simulink model "Xcvr_SSB_AM_2p5"  (Simulink 7.4)
settings: Solver=VariableStepDiscrete  SolverMode=SingleTasking  StartTime=0.0  StopTime=10  RelTol=1e-3
PreLoadFcn:
  | Fs=80e6;
  | 
  | phee=da_rom();
  | [phee_1,phee_2]=da_i2_rom();
  | 
  | Dcic=64;       % CIC decimation
  | Dfac=128;    % following DA filter decimation
  | N = 6;           %       (2^(N+1))=Dfac
  | Daudio=Dcic*Dfac;
  | Faudio=Fs/Daudio;
  | 
  | load info_filt_ssb_4
  | load Serial_Intfc_Stream_5
  | 
  | % AGC related
  | x=0.5:1/256:(1-1/256);
  | addr=(x-0.5)*256;
  | y=1./x;
undefined symbols (not defined in the file): Serial_Interface, ssb_coef, xlipgetpartsetting
libraries: xbsIndex_r4 x1305, dspsrcs4 x5, simulink x2, dspsigops x2, dspsnks4 x1
(part 7 of 11)

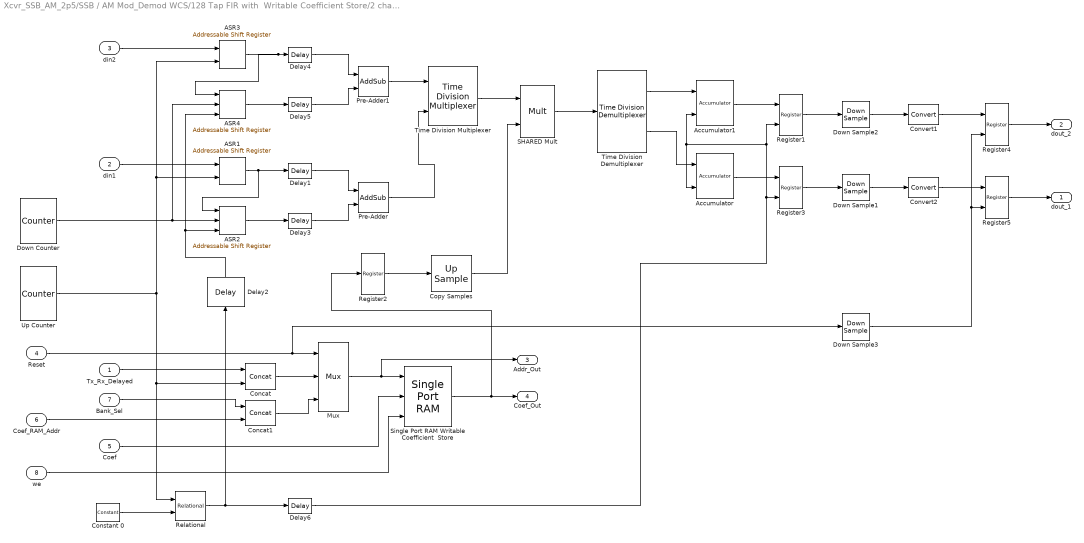
== system Xcvr_SSB_AM_2p5/SSB / AM Mod_Demod WCS/128 Tap FIR with  Writable Coefficient Store/2 channel (IQ)  SHARED MPY MAC with Writable Coefficient Store ==
  Tx_Rx_Delayed : Inport  OutDataType=sfix(16)  OutScaling=2^0
  din1 : Inport  Port=2  OutDataType=sfix(16)  OutScaling=2^0
  din2 : Inport  Port=3  OutDataType=sfix(16)  OutScaling=2^0
  Reset : Inport  Port=4  OutDataType=sfix(16)  OutScaling=2^0
  Coef : Inport  Port=5  OutDataType=sfix(16)  OutScaling=2^0
  Coef_RAM_Addr : Inport  Port=6  OutDataType=sfix(16)  OutScaling=2^0
  Bank_Sel : Inport  Port=7  OutDataType=sfix(16)  OutScaling=2^0
  we : Inport  Port=8  OutDataType=sfix(16)  OutScaling=2^0
  ASR1 : xbsIndex_r4/Addressable Shift Register  infer_latency=on  depth=2  initVector=0  en=off  dbl_ovrd=off  use_behavioral_HDL=off  use_rpm=off  block_type=addrsr
      settings: infoedit="Delay of configurable length.  Any element in the delay line can be addressed and driven onto the output port.<P><P>Hardware notes: Implemented using SRL16s.  If a Virtex-II device is used, multiple SRLC16s are cascaded together."  xl_area=[0, 0, 0, 0, 0, 0, 0]  block_version=VER_STRING_GOES_HERE
  ASR2 : xbsIndex_r4/Addressable Shift Register  infer_latency=on  depth=2  initVector=0  en=on  dbl_ovrd=off  use_behavioral_HDL=off  use_rpm=off  block_type=addrsr
      settings: infoedit="Delay of configurable length.  Any element in the delay line can be addressed and driven onto the output port.<P><P>Hardware notes: Implemented using SRL16s.  If a Virtex-II device is used, multiple SRLC16s are cascaded together."  xl_area=[0, 0, 0, 0, 0, 0, 0]  block_version=VER_STRING_GOES_HERE
  ASR3 : xbsIndex_r4/Addressable Shift Register  infer_latency=on  depth=2  initVector=0  en=off  dbl_ovrd=off  use_behavioral_HDL=off  use_rpm=off  block_type=addrsr
      settings: infoedit="Delay of configurable length.  Any element in the delay line can be addressed and driven onto the output port.<P><P>Hardware notes: Implemented using SRL16s.  If a Virtex-II device is used, multiple SRLC16s are cascaded together."  xl_area=[0, 0, 0, 0, 0, 0, 0]  block_version=VER_STRING_GOES_HERE
  ASR4 : xbsIndex_r4/Addressable Shift Register  infer_latency=on  depth=2  initVector=0  en=on  dbl_ovrd=off  use_behavioral_HDL=off  use_rpm=off  block_type=addrsr
      settings: infoedit="Delay of configurable length.  Any element in the delay line can be addressed and driven onto the output port.<P><P>Hardware notes: Implemented using SRL16s.  If a Virtex-II device is used, multiple SRLC16s are cascaded together."  xl_area=[0, 0, 0, 0, 0, 0, 0]  block_version=VER_STRING_GOES_HERE
  Accumulator : xbsIndex_r4/Accumulator  operation=Add  n_bits=ceil(log2(max(1,sum(abs(coef*2^coef_bin_pt)))))+smpl_n_bits + 1  overflow=Wrap  scale=1  rst=on  hasbypass=on  en=off  dbl_ovrd=off  use_behavioral_HDL=on  implementation=Fabric  block_type=accum
      settings: infoedit="Adder or subtractor-based accumulator.   Output type and binary point position match the input.<P><P>Hardware notes: When \"Reinitialize with Input 'b' on Reset\" is selected, the accumulator is forced to run at the system rate even if the input 'b' is running at a slower rate."  xl_area=[0, 0, 0, 0, 0, 0, 0]  block_version=VER_STRING_GOES_HERE
  Accumulator1 : xbsIndex_r4/Accumulator  operation=Add  n_bits=ceil(log2(max(1,sum(abs(coef*2^coef_bin_pt)))))+smpl_n_bits + 1  overflow=Wrap  scale=1  rst=on  hasbypass=on  en=off  dbl_ovrd=off  use_behavioral_HDL=on  implementation=Fabric  block_type=accum
      settings: infoedit="Adder or subtractor-based accumulator.   Output type and binary point position match the input.<P><P>Hardware notes: When \"Reinitialize with Input 'b' on Reset\" is selected, the accumulator is forced to run at the system rate even if the input 'b' is running at a slower rate."  xl_area=[0, 0, 0, 0, 0, 0, 0]  block_version=VER_STRING_GOES_HERE
  Concat : xbsIndex_r4/Concat  num_inputs=2  dbl_ovrd=off  block_type=concat
      settings: block_version=12.2
  Concat1 : xbsIndex_r4/Concat  num_inputs=2  dbl_ovrd=off  block_type=concat
      settings: block_version=12.2
  Constant 0 : xbsIndex_r4/Constant  arith_type=Unsigned  const=0  n_bits=1  bin_pt=0  explicit_period=off  period=1  equ=P=C  opselect=C  inp2=PCIN>>17  opr=+  inp1=P  carry=CIN  dbl_ovrd=off  block_type=constant
      settings: block_version=VER_STRING_GOES_HERE
  Convert1 : xbsIndex_r4/Convert  arith_type="Signed  (2's comp)"  n_bits=18  bin_pt=17  quantization="Round  (unbiased: +/- Inf)"  overflow=Wrap  en=off  latency=0  dbl_ovrd=off  pipeline=off  block_type=convert
      settings: block_version=9.2.00
  Convert2 : xbsIndex_r4/Convert  arith_type="Signed  (2's comp)"  n_bits=18  bin_pt=17  quantization="Round  (unbiased: +/- Inf)"  overflow=Wrap  en=off  latency=0  dbl_ovrd=off  pipeline=off  block_type=convert
      settings: block_version=9.2.00
  Copy Samples : xbsIndex_r4/Up Sample  sample_ratio=2  copy_samples=on  en=off  latency=0  dbl_ovrd=off  block_type=usamp
      settings: block_version=12.1
  Delay{1,3..5} (4 alike) : xbsIndex_r4/Delay  en=off  latency=1  dbl_ovrd=off  reg_retiming=off  block_type=delay
      settings: infoedit="Delay line having  configurable length.<P><P>Hardware notes: A delay line is a chain, each link of which is an SRL16 followed by a flip-flop. If register retiming is enabled, the delay line is a chain of flip-flops."  xl_area=[0, 0, 0, 0, 0, 0, 0]  block_version=VER_STRING_GOES_HERE
  Delay2 : xbsIndex_r4/Delay  en=off  latency=(length(coef)/2)-2  dbl_ovrd=off  reg_retiming=off  block_type=delay
      settings: infoedit="Delay line having  configurable length.<P><P>Hardware notes: A delay line is a chain, each link of which is an SRL16 followed by a flip-flop. If register retiming is enabled, the delay line is a chain of flip-flops."  xl_area=[0, 0, 0, 0, 0, 0, 0]  block_version=VER_STRING_GOES_HERE
  Delay6 : xbsIndex_r4/Delay  en=off  latency=3  dbl_ovrd=off  reg_retiming=off  block_type=delay
      settings: xl_area=[0, 0, 0, 0, 0, 0, 0]  block_version=VER_STRING_GOES_HERE
  Down Counter : xbsIndex_r4/Counter  cnt_type=Count Limited  cnt_to=0  operation=Down  start_count=(length(coef)/2)-1  cnt_by_val=1  arith_type=Unsigned  n_bits=ceil(log2(length(coef)/2))  bin_pt=0  load_pin=off  rst=off  en=off  explicit_period=on  period=smpl_period/(length(coef)/2)  dbl_ovrd=off  use_behavioral_HDL=off  implementation=Fabric  use_rpm=off  block_type=counter
      settings: xl_area=[0, 0, 0, 0, 0, 0, 0]  block_version=VER_STRING_GOES_HERE
  Down Sample1 : xbsIndex_r4/Down Sample  sample_ratio=length(coef)/2  sample_phase="Last Value of Frame  (most efficient)"  en=off  latency=1  dbl_ovrd=off  block_type=dsamp
      settings: xl_area=[0, 0, 0, 0, 0, 0, 0]  block_version=VER_STRING_GOES_HERE
  Down Sample2 : xbsIndex_r4/Down Sample  sample_ratio=length(coef)/2  sample_phase="Last Value of Frame  (most efficient)"  en=off  latency=1  dbl_ovrd=off  block_type=dsamp
      settings: xl_area=[0, 0, 0, 0, 0, 0, 0]  block_version=VER_STRING_GOES_HERE
  Down Sample3 : xbsIndex_r4/Down Sample  sample_ratio=4  sample_phase="Last Value of Frame  (most efficient)"  en=off  latency=1  dbl_ovrd=off  block_type=dsamp
      settings: xl_area=[0, 0, 0, 0, 0, 0, 0]  block_version=VER_STRING_GOES_HERE
  Mux : xbsIndex_r4/Mux  inputs=2  en=off  latency=0  precision=Full  arith_type=Unsigned  n_bits=16  bin_pt=14  quantization=Truncate  overflow=Wrap  dbl_ovrd=off  block_type=mux
      settings: block_version=12.1
  Pre-Adder : xbsIndex_r4/AddSub  mode=Addition  use_carryin=off  use_carryout=off  en=off  latency=1  precision=Full  arith_type=Unsigned  n_bits=8  bin_pt=2  quantization=Truncate  overflow=Wrap  dbl_ovrd=off  use_behavioral_HDL=on  hw_selection=Fabric  pipelined=off  use_rpm=off  block_type=addsub
      settings: xl_area=[0, 0, 0, 0, 0, 0, 0]  block_version=VER_STRING_GOES_HERE
  Pre-Adder1 : xbsIndex_r4/AddSub  mode=Addition  use_carryin=off  use_carryout=off  en=off  latency=1  precision=Full  arith_type=Unsigned  n_bits=8  bin_pt=2  quantization=Truncate  overflow=Wrap  dbl_ovrd=off  use_behavioral_HDL=on  hw_selection=Fabric  pipelined=off  use_rpm=off  block_type=addsub
      settings: xl_area=[0, 0, 0, 0, 0, 0, 0]  block_version=VER_STRING_GOES_HERE
  Register1 : xbsIndex_r4/Register  init=0  rst=off  en=on  dbl_ovrd=off  block_type=register
      settings: xl_area=[0, 0, 0, 0, 0, 0, 0]  block_version=VER_STRING_GOES_HERE
  Register2 : xbsIndex_r4/Register  init=0  rst=off  en=off  dbl_ovrd=off  block_type=register
      settings: xl_area=[0, 0, 0, 0, 0, 0, 0]  block_version=VER_STRING_GOES_HERE
  Register3 : xbsIndex_r4/Register  init=0  rst=off  en=on  dbl_ovrd=off  block_type=register
      settings: xl_area=[0, 0, 0, 0, 0, 0, 0]  block_version=VER_STRING_GOES_HERE
  Register4 : xbsIndex_r4/Register  init=0  rst=on  en=off  dbl_ovrd=off  block_type=register
      settings: xl_area=[0, 0, 0, 0, 0, 0, 0]  block_version=VER_STRING_GOES_HERE
  Register5 : xbsIndex_r4/Register  init=0  rst=on  en=off  dbl_ovrd=off  block_type=register
      settings: xl_area=[0, 0, 0, 0, 0, 0, 0]  block_version=VER_STRING_GOES_HERE
  Relational : xbsIndex_r4/Relational  mode=a=b  en=off  latency=1  dbl_ovrd=off  block_type=relational
      settings: xl_area=[0, 0, 0, 0, 0, 0, 0]  block_version=VER_STRING_GOES_HERE
  SHARED Mult : xbsIndex_r4/Mult  precision=User Defined  arith_type="Signed  (2's comp)"  n_bits=max(ceil(log2(max(1,max(abs(coef*2^coef_bin_pt)))))+smpl_n_bits + 1,smpl_bin_pt+coef_bin_pt)  bin_pt=smpl_bin_pt+coef_bin_pt  quantization="Round  (unbiased: +/- Inf)"  overflow=Wrap  en=off  latency=2  dbl_ovrd=off  use_behavioral_HDL=off  opt=Speed  use_embedded=on  optimum_pipeline=off  pipeline=on  use_rpm=on  placement_style=Rectangular shape  block_type=mult
      settings: infoedit=Multiplies two values.<P><P>Hardware notes: To use the internal pipeline stage of the dedicated multiplier you must select 'Pipeline to Greatest Extent Possible'.  xl_area=[0, 0, 0, 0, 0, 0, 0]  block_version=VER_STRING_GOES_HERE
  Single Port RAM Writable Coefficient  Store : xbsIndex_r4/Single Port RAM  depth=length(coef)  initVector=horzcat(coef(1:(length(coef)/2)),coef(1:(length(coef)/2)))  distributed_mem=Block RAM  write_mode=No Read On Write  rst=off  init_reg=0  en=off  latency=1  dbl_ovrd=off  optimize=Area  use_rpm=on  block_type=spram
      settings: block_version=12.1
  Time Division Demultiplexer : xbsIndex_r4/Time Division Demultiplexer  frame_pattern=[1 1]  impl_style=Multiple Channel  vin=off  dbl_ovrd=off  explicit_period=off  period=1  block_type=tdd
      settings: infoedit=Samples presented at the input are selected and down-sampled according to the frame sampling pattern specified. The sampled input is presented either as a single or multiple channel at the output.  block_version=12.1
  Time Division Multiplexer : xbsIndex_r4/Time Division Multiplexer  inputs=2  vin=off  dbl_ovrd=off  explicit_period=off  period=1  block_type=tdm
      settings: infoedit="Multiple inputs are sampled and  presented serially at the output."  block_version=12.1
  Up Counter : xbsIndex_r4/Counter  cnt_type=Count Limited  cnt_to=(length(coef)/2)-1  operation=Up  start_count=0  cnt_by_val=1  arith_type=Unsigned  n_bits=ceil(log2(length(coef)/2))  bin_pt=0  load_pin=off  rst=off  en=off  explicit_period=on  period=smpl_period/(length(coef)/2)  dbl_ovrd=off  use_behavioral_HDL=off  implementation=Fabric  use_rpm=off  block_type=counter
      settings: xl_area=[0, 0, 0, 0, 0, 0, 0]  block_version=VER_STRING_GOES_HERE
  dout_1 : Outport  OutDataType=sfix(16)  OutScaling=2^0
  dout_2 : Outport  Port=2  OutDataType=sfix(16)  OutScaling=2^0
  Addr_Out : Outport  Port=3  OutDataType=sfix(16)  OutScaling=2^0
  Coef_Out : Outport  Port=4  OutDataType=sfix(16)  OutScaling=2^0
  wires:
  Down Counter/1 -> ASR2/2, ASR4/2
  Delay2/1 -> ASR2/3, ASR4/3
  Pre-Adder/1 -> Time Division Multiplexer/2
  Delay3/1 -> Pre-Adder/2
  ASR2/1 -> Delay3/1
  Register3/1 -> Down Sample1/1
  Delay1/1 -> Pre-Adder/1
  ASR1/1 -> ASR2/1, Delay1/1
  Up Counter/1 -> ASR1/2, ASR3/2, Relational/1, Concat/2
  din1/1 -> ASR1/1
  Down Sample1/1 -> Convert2/1
  Constant 0/1 -> Relational/2
  Relational/1 -> Delay6/1, Delay2/1
  Register2/1 -> Copy Samples/1
  Delay5/1 -> Pre-Adder1/2
  Delay4/1 -> Pre-Adder1/1
  ASR3/1 -> ASR4/1, Delay4/1
  din2/1 -> ASR3/1
  Pre-Adder1/1 -> Time Division Multiplexer/1
  Register1/1 -> Down Sample2/1
  Down Sample2/1 -> Convert1/1
  ASR4/1 -> Delay5/1
  Time Division Multiplexer/1 -> SHARED Mult/1
  SHARED Mult/1 -> Time Division Demultiplexer/1
  Accumulator/1 -> Register3/1
  Time Division Demultiplexer/2 -> Accumulator/1
  Time Division Demultiplexer/1 -> Accumulator1/1
  Accumulator1/1 -> Register1/1
  Delay6/1 -> Register3/2, Register1/2, Accumulator1/2, Accumulator/2
  Copy Samples/1 -> SHARED Mult/2
  Mux/1 -> Addr_Out/1, Single Port RAM Writable Coefficient  Store/1
  Coef/1 -> Single Port RAM Writable Coefficient  Store/2
  we/1 -> Single Port RAM Writable Coefficient  Store/3
  Single Port RAM Writable Coefficient  Store/1 -> Coef_Out/1, Register2/1
  Reset/1 -> Mux/1, Down Sample3/1
  Convert1/1 -> Register4/1
  Register4/1 -> dout_2/1
  Convert2/1 -> Register5/1
  Register5/1 -> dout_1/1
  Down Sample3/1 -> Register5/2, Register4/2
  Concat/1 -> Mux/2
  Tx_Rx_Delayed/1 -> Concat/1
  Concat1/1 -> Mux/3
  Coef_RAM_Addr/1 -> Concat1/2
  Bank_Sel/1 -> Concat1/1

== system Xcvr_SSB_AM_2p5/SSB / AM Mod_Demod WCS/128 Tap FIR with  Writable Coefficient Store/Information_Filter_Transient_Suppressor ==
  note: W1QG:  This is a desparate HACK.
      |
      | The right way to do this would be to have separate sample memory in the
      | information filter for RX and TX.
      |
      | However, this would double the storage from 256 16 bit words to 256.
      | It might fit, then again, it might not.  Try this first.
  note: On RX, supress filter output to TX DA / CIC interpolation filter input to load it with zeros.
      | On transition fom RX to TX, continue to suppress for N more samples to allow
      | information filter output to forget the previous Rx data it had in its mind.
      | N =Info Filter length (128) plus 2 more for good measure
  note: (k6jca note:  in attempt to remove an RX glitch when transitioning from
      | Tx to Rx in AM mode, I've added "Supress_Rx_while_Tx" to Dick's original circuit.
      | But I don't do an additional "Load Zeroes", as I am not sure there's a need for it,
      | if we are also suppressing the filter's output.)
  Tx_Rx_Delayed : Inport  OutDataType=fixdt(1, 16)  OutScaling=2^0
  Constant : xbsIndex_r4/Constant  arith_type=Boolean  const=0  n_bits=16  bin_pt=14  explicit_period=off  period=1  equ=P=C  opselect=C  inp2=PCIN>>17  opr=+  inp1=P  carry=CIN  dbl_ovrd=off  block_type=constant
      settings: block_version=12.2
  Delay : xbsIndex_r4/Delay  en=off  latency=1  dbl_ovrd=off  reg_retiming=off  block_type=delay
      settings: block_version=12.1
  Inverter1 : xbsIndex_r4/Inverter  en=off  latency=0  dbl_ovrd=off  block_type=inv
      settings: block_version=12.1
  Inverter2 : xbsIndex_r4/Inverter  en=off  latency=0  dbl_ovrd=off  block_type=inv
      settings: block_version=12.1
  Logical : xbsIndex_r4/Logical  logical_function=XOR  inputs=2  en=off  latency=0  precision=Full  arith_type=Unsigned  n_bits=16  bin_pt=0  align_bp=on  dbl_ovrd=off  block_type=logical
      settings: block_version=12.1
  Logical1 : xbsIndex_r4/Logical  logical_function=AND  inputs=2  en=off  latency=0  precision=Full  arith_type=Unsigned  n_bits=16  bin_pt=0  align_bp=on  dbl_ovrd=off  block_type=logical
      settings: block_version=12.1
  Logical2 : xbsIndex_r4/Logical  logical_function=AND  inputs=2  en=off  latency=0  precision=Full  arith_type=Unsigned  n_bits=16  bin_pt=0  align_bp=on  dbl_ovrd=off  block_type=logical
      settings: block_version=12.1
  Logical3 : xbsIndex_r4/Logical  logical_function=OR  inputs=2  en=off  latency=0  precision=Full  arith_type=Unsigned  n_bits=16  bin_pt=0  align_bp=on  dbl_ovrd=off  block_type=logical
      settings: block_version=12.1
  Logical4 : xbsIndex_r4/Logical  logical_function=OR  inputs=2  en=off  latency=0  precision=Full  arith_type=Unsigned  n_bits=16  bin_pt=0  align_bp=on  dbl_ovrd=off  block_type=logical
      settings: block_version=12.1
  N_Sample_One_Shot : Subsystem  mask{N=128+2}
      mask prompts: N "N=   (2<N<=255)"
  Supress_Tx_while_Rx : Outport  OutDataType=fixdt(1, 16)  OutScaling=2^0
  Supress_Rx_while_Tx : Outport  Port=2  OutDataType=fixdt(1, 16)  OutScaling=2^0
  Load Zeros : Outport  Port=3  OutDataType=fixdt(1, 16)  OutScaling=2^0
  wires:
  Tx_Rx_Delayed/1 -> Delay/1, Logical1/2, Inverter2/1, Logical/1, Inverter1/1
  Delay/1 -> Logical/2
  Logical/1 -> N_Sample_One_Shot/1(In)  "Rx_to_Tx"
  Logical3/1 -> Supress_Tx_while_Rx/1
  Inverter2/1 -> Logical2/1
  N_Sample_One_Shot/1(Out) -> Logical1/1, Logical2/2
  Logical1/1 -> Load Zeros/1, Logical3/2
  Logical2/1 -> Logical4/1
  Logical4/1 -> Supress_Rx_while_Tx/1
  Inverter1/1 -> Logical3/1
  Constant/1 -> Logical4/2

== system Xcvr_SSB_AM_2p5/SSB / AM Mod_Demod WCS/Sequential_Complex_abs()/Iterative SQRT ==
  Xin : Inport
  Run : Inport  Port=2
  From SQR : Inport  Port=3
  AddSub : xbsIndex_r4/AddSub  mode=Addition  use_carryin=off  use_carryout=off  en=off  latency=0  precision=User Defined  arith_type=Unsigned  n_bits=32  bin_pt=31  quantization=Truncate  overflow=Wrap  dbl_ovrd=off  use_behavioral_HDL=off  hw_selection=Fabric  pipelined=off  block_type=addsub
      settings: block_version=12.1
  AddSub1 : xbsIndex_r4/AddSub  mode=Subtraction  use_carryin=off  use_carryout=off  en=off  latency=0  precision=User Defined  arith_type="Signed  (2's comp)"  n_bits=32  bin_pt=31  quantization=Truncate  overflow=Wrap  dbl_ovrd=off  use_behavioral_HDL=off  hw_selection=Fabric  pipelined=off  block_type=addsub
      settings: block_version=12.1
  Constant1 : xbsIndex_r4/Constant  arith_type=Unsigned  const=1/32  n_bits=32  bin_pt=31  explicit_period=off  period=1  equ=P=C  opselect=C  inp2=PCIN>>17  opr=+  inp1=P  carry=CIN  dbl_ovrd=off  block_type=constant
      settings: block_version=12.1
  Down Sample : xbsIndex_r4/Down Sample  sample_ratio=32  sample_phase="Last Value of Frame  (most efficient)"  en=off  latency=1  dbl_ovrd=off  block_type=dsamp
      settings: block_version=12.1
  Inverter : xbsIndex_r4/Inverter  en=off  latency=0  dbl_ovrd=off  block_type=inv
      settings: block_version=12.1
  Logical : xbsIndex_r4/Logical  logical_function=AND  inputs=2  en=off  latency=0  precision=Full  arith_type=Unsigned  n_bits=16  bin_pt=0  align_bp=on  dbl_ovrd=off  block_type=logical
      settings: block_version=12.1
  Mux : xbsIndex_r4/Mux  inputs=2  en=off  latency=0  precision=Full  arith_type=Unsigned  n_bits=16  bin_pt=14  quantization=Truncate  overflow=Wrap  dbl_ovrd=off  block_type=mux
      settings: block_version=12.1
  Register : xbsIndex_r4/Register  init=0  rst=off  en=on  dbl_ovrd=off  block_type=register
      settings: block_version=12.1
  Register1 : xbsIndex_r4/Register  init=0  rst=off  en=off  dbl_ovrd=off  block_type=register
      settings: block_version=12.1
  Raw Sqrt Out : Outport
  "To SQR " : Outport  Port=2
  wires:
  Mux/1 -> Register/1, "To SQR "/1
  Constant1/1 -> Mux/3
  AddSub/1 -> Mux/2
  Register/1 -> AddSub/1, Down Sample/1
  AddSub1/1 -> AddSub/2  "Error"
  Xin/1 -> AddSub1/1
  From SQR/1 -> AddSub1/2
  Register1/1 -> Inverter/1
  Inverter/1 -> Logical/2
  Run/1 -> Logical/1, Register1/1, Register/2
  Logical/1 -> Mux/1
  Down Sample/1 -> Raw Sqrt Out/1

== system Xcvr_SSB_AM_2p5/SSB / AM Mod_Demod WCS/Sequential_Complex_abs()/Pre Scaler ==
  X : Inport
  AddSub : xbsIndex_r4/AddSub  mode=Addition  use_carryin=off  use_carryout=off  en=off  latency=0  precision=User Defined  arith_type=Unsigned  n_bits=4  bin_pt=0  quantization=Truncate  overflow=Wrap  dbl_ovrd=off  use_behavioral_HDL=off  hw_selection=Fabric  pipelined=off  block_type=addsub
      settings: block_version=12.1
  Constant : xbsIndex_r4/Constant  arith_type=Unsigned  const=0  n_bits=5  bin_pt=0  explicit_period=off  period=1  equ=P=C  opselect=C  inp2=PCIN>>17  opr=+  inp1=P  carry=CIN  dbl_ovrd=off  block_type=constant
      settings: block_version=12.1
  Constant1 : xbsIndex_r4/Constant  arith_type=Boolean  const=1  n_bits=5  bin_pt=0  explicit_period=off  period=1  equ=P=C  opselect=C  inp2=PCIN>>17  opr=+  inp1=P  carry=CIN  dbl_ovrd=off  block_type=constant
      settings: block_version=12.1
  Constant2 : xbsIndex_r4/Constant  arith_type=Unsigned  const=0.25  n_bits=32  bin_pt=31  explicit_period=off  period=1  equ=P=C  opselect=C  inp2=PCIN>>17  opr=+  inp1=P  carry=CIN  dbl_ovrd=off  block_type=constant
      settings: block_version=12.1
  Constant3 : xbsIndex_r4/Constant  arith_type=Unsigned  const=1  n_bits=4  bin_pt=0  explicit_period=on  period=1/(32*Faudio)  equ=P=C  opselect=C  inp2=PCIN>>17  opr=+  inp1=P  carry=CIN  dbl_ovrd=off  block_type=constant
      settings: block_version=12.1
  Counter : xbsIndex_r4/Counter  cnt_type=Free Running  cnt_to=Inf  operation=Up  start_count=0  cnt_by_val=1  arith_type=Unsigned  n_bits=5  bin_pt=0  load_pin=off  rst=off  en=off  explicit_period=on  period=1/(32*Faudio)  dbl_ovrd=off  use_behavioral_HDL=off  implementation=Fabric  block_type=counter
      settings: block_version=12.1
  Inverter : xbsIndex_r4/Inverter  en=off  latency=0  dbl_ovrd=off  block_type=inv
      settings: block_version=12.1
  Mux : xbsIndex_r4/Mux  inputs=2  en=off  latency=0  precision=Full  arith_type=Unsigned  n_bits=16  bin_pt=14  quantization=Truncate  overflow=Wrap  dbl_ovrd=off  block_type=mux
      settings: block_version=12.1
  Mux1 : xbsIndex_r4/Mux  inputs=2  en=off  latency=0  precision=Full  arith_type=Unsigned  n_bits=16  bin_pt=14  quantization=Truncate  overflow=Wrap  dbl_ovrd=off  block_type=mux
      settings: block_version=12.1
  Register : xbsIndex_r4/Register  init=0  rst=on  en=on  dbl_ovrd=off  block_type=register
      settings: block_version=12.1
  Register1 : xbsIndex_r4/Register  init=0  rst=off  en=on  dbl_ovrd=off  block_type=register
      settings: block_version=12.1
  Relational : xbsIndex_r4/Relational  mode=a=b  en=off  latency=0  dbl_ovrd=off  block_type=relational
      settings: block_version=12.1
  Relational1 : xbsIndex_r4/Relational  mode=a<=b  en=off  latency=0  dbl_ovrd=off  block_type=relational
      settings: block_version=12.1
  Shift : xbsIndex_r4/Shift  shift_dir=Left  shift_bits=2  en=off  latency=0  precision=Full  arith_type="Signed  (2's comp)"  n_bits=16  bin_pt=14  quantization=Truncate  overflow=Wrap  dbl_ovrd=off  block_type=shift
      settings: block_version=12.1
  X*(2^2n) : Outport
  Done : Outport  Port=2
  Shift Count : Outport  Port=3
  wires:
  Mux/1 -> Register1/1
  Counter/1 -> Relational/1
  Constant/1 -> Relational/2
  Relational/1 -> Mux/1, Mux1/1, Register/2
  Register1/1 -> Relational1/1, Shift/1, X*(2^2n)/1
  Shift/1 -> Mux/2
  X/1 -> Mux/3
  Mux1/1 -> Register1/2
  Constant1/1 -> Mux1/3
  Relational1/1 -> Mux1/2, Register/3, Inverter/1
  Constant2/1 -> Relational1/2
  AddSub/1 -> Register/1
  Inverter/1 -> Done/1
  Register/1 -> AddSub/1, Shift Count/1
  Constant3/1 -> AddSub/2

== system Xcvr_SSB_AM_2p5/SSB / AM Mod_Demod WCS/Sequential_Complex_abs()/Sequential Post Scale ==
  X : Inport
  n : Inport  Port=2
  Constant : xbsIndex_r4/Constant  arith_type=Unsigned  const=0  n_bits=5  bin_pt=0  explicit_period=off  period=1  equ=P=C  opselect=C  inp2=PCIN>>17  opr=+  inp1=P  carry=CIN  dbl_ovrd=off  block_type=constant
      settings: block_version=12.1
  Constant1 : xbsIndex_r4/Constant  arith_type=Boolean  const=1  n_bits=5  bin_pt=0  explicit_period=off  period=1  equ=P=C  opselect=C  inp2=PCIN>>17  opr=+  inp1=P  carry=CIN  dbl_ovrd=off  block_type=constant
      settings: block_version=12.1
  Counter : xbsIndex_r4/Counter  cnt_type=Free Running  cnt_to=Inf  operation=Up  start_count=0  cnt_by_val=1  arith_type=Unsigned  n_bits=4  bin_pt=0  load_pin=off  rst=off  en=off  explicit_period=on  period=1/(16*Faudio)  dbl_ovrd=off  use_behavioral_HDL=off  implementation=Fabric  block_type=counter
      settings: block_version=12.1
  Down Sample : xbsIndex_r4/Down Sample  sample_ratio=16  sample_phase="Last Value of Frame  (most efficient)"  en=off  latency=1  dbl_ovrd=off  block_type=dsamp
      settings: block_version=12.1
  Inverter : xbsIndex_r4/Inverter  en=off  latency=0  dbl_ovrd=off  block_type=inv
      settings: block_version=12.1
  Mux : xbsIndex_r4/Mux  inputs=2  en=off  latency=0  precision=Full  arith_type=Unsigned  n_bits=16  bin_pt=14  quantization=Truncate  overflow=Wrap  dbl_ovrd=off  block_type=mux
      settings: block_version=12.1
  Mux1 : xbsIndex_r4/Mux  inputs=2  en=off  latency=0  precision=Full  arith_type=Unsigned  n_bits=16  bin_pt=14  quantization=Truncate  overflow=Wrap  dbl_ovrd=off  block_type=mux
      settings: block_version=12.1
  Register1 : xbsIndex_r4/Register  init=0  rst=off  en=on  dbl_ovrd=off  block_type=register
      settings: block_version=12.1
  Relational : xbsIndex_r4/Relational  mode=a=b  en=off  latency=0  dbl_ovrd=off  block_type=relational
      settings: block_version=12.1
  Relational1 : xbsIndex_r4/Relational  mode=a>b  en=off  latency=0  dbl_ovrd=off  block_type=relational
      settings: block_version=12.1
  Shift : xbsIndex_r4/Shift  shift_dir=Right  shift_bits=1  en=off  latency=0  precision=Full  arith_type="Signed  (2's comp)"  n_bits=16  bin_pt=14  quantization=Truncate  overflow=Wrap  dbl_ovrd=off  block_type=shift
      settings: block_version=12.1
  Up Sample : xbsIndex_r4/Up Sample  sample_ratio=16  copy_samples=on  en=off  latency=0  dbl_ovrd=off  block_type=usamp
      settings: block_version=12.1
  Up Sample1 : xbsIndex_r4/Up Sample  sample_ratio=16  copy_samples=on  en=off  latency=0  dbl_ovrd=off  block_type=usamp
      settings: block_version=12.1
  X*(2^-n) : Outport
  wires:
  Inverter/1 -> Mux1/2
  Constant1/1 -> Mux1/3
  Mux1/1 -> Register1/2
  X/1 -> Up Sample/1
  Shift/1 -> Mux/2
  Register1/1 -> Shift/1, Down Sample/1
  Relational/1 -> Mux1/1, Mux/1
  Constant/1 -> Relational/2
  Counter/1 -> Relational/1, Relational1/1
  Mux/1 -> Register1/1
  n/1 -> Up Sample1/1
  Relational1/1 -> Inverter/1
  Up Sample/1 -> Mux/3
  Up Sample1/1 -> Relational1/2
  Down Sample/1 -> X*(2^-n)/1

== system Xcvr_SSB_AM_2p5/SSB / AM Mod_Demod WCS/Sequential_Complex_abs()/Time Shared Square Operator ==
  A : Inport
  B : Inport  Port=2
  C : Inport  Port=3
  Mult : xbsIndex_r4/Mult  precision=User Defined  arith_type=Unsigned  n_bits=32  bin_pt=31  quantization=Truncate  overflow=Saturate  en=off  latency=0  dbl_ovrd=off  use_behavioral_HDL=off  opt=Speed  use_embedded=on  optimum_pipeline=off  pipeline=on  use_rpm=on  placement_style=Triangular  block_type=mult
      settings: block_version=12.1
  Terminator : Terminator
  Time Division Demultiplexer : xbsIndex_r4/Time Division Demultiplexer  frame_pattern=[1 1 1 1]  impl_style=Multiple Channel  vin=off  dbl_ovrd=off  explicit_period=off  period=1  block_type=tdd
      settings: infoedit=Samples presented at the input are selected and down-sampled according to the frame sampling pattern specified. The sampled input is presented either as a single or multiple channel at the output.  block_version=12.1
  Time Division Multiplexer : xbsIndex_r4/Time Division Multiplexer  inputs=4  vin=off  dbl_ovrd=off  explicit_period=off  period=1  block_type=tdm
      settings: infoedit="Multiple inputs are sampled and  presented serially at the output."  block_version=12.1
  A^2 : Outport
  B^2 : Outport  Port=2
  C^2 : Outport  Port=3
  wires:
  A/1 -> Time Division Multiplexer/1
  B/1 -> Time Division Multiplexer/2
  C/1 -> Time Division Multiplexer/3, Time Division Multiplexer/4
  Time Division Multiplexer/1 -> Mult/1, Mult/2
  Mult/1 -> Time Division Demultiplexer/1
  Time Division Demultiplexer/3 -> C^2/1
  Time Division Demultiplexer/2 -> B^2/1
  Time Division Demultiplexer/1 -> A^2/1
  Time Division Demultiplexer/4 -> Terminator/1

== system Xcvr_SSB_AM_2p5/Serial Interface1/Interrupt_Generator/IRPT_REG0 ==
  DIN : Inport  OutDataType=fixdt(1, 16)  OutScaling=2^0
  EN_IRPT : Inport  Port=2  OutDataType=fixdt(1, 16)  OutScaling=2^0
  CLR_IRPT : Inport  Port=3  OutDataType=fixdt(1, 16)  OutScaling=2^0
  Delay : xbsIndex_r4/Delay  en=off  latency=1  dbl_ovrd=off  reg_retiming=off  block_type=delay
      settings: block_version=12.1
  Logical1 : xbsIndex_r4/Logical  logical_function=OR  inputs=2  en=off  latency=0  precision=Full  arith_type=Unsigned  n_bits=16  bin_pt=0  align_bp=on  dbl_ovrd=off  block_type=logical
      settings: block_version=12.1
  Logical2 : xbsIndex_r4/Logical  logical_function=XOR  inputs=2  en=off  latency=0  precision=Full  arith_type=Unsigned  n_bits=16  bin_pt=0  align_bp=on  dbl_ovrd=off  block_type=logical
      settings: block_version=12.1
  Logical4 : xbsIndex_r4/Logical  logical_function=AND  inputs=2  en=off  latency=0  precision=Full  arith_type=Unsigned  n_bits=16  bin_pt=0  align_bp=on  dbl_ovrd=off  block_type=logical
      settings: block_version=12.1
  Register : xbsIndex_r4/Register  init=0  rst=on  en=off  dbl_ovrd=off  block_type=register
      settings: block_version=12.1
  IRPT_OUT : Outport  OutDataType=fixdt(1, 16)  OutScaling=2^0
  wires:
  Delay/1 -> Logical2/2
  DIN/1 -> Delay/1, Logical2/1
  Logical2/1 -> Logical4/1
  EN_IRPT/1 -> Logical4/2
  Logical4/1 -> Logical1/2
  Logical1/1 -> Register/1
  Register/1 -> IRPT_OUT/1, Logical1/1
  CLR_IRPT/1 -> Register/2

== system Xcvr_SSB_AM_2p5/Serial Interface1/Interrupt_Generator/IRPT_REG1 ==
  DIN : Inport  OutDataType=fixdt(1, 16)  OutScaling=2^0
  EN_IRPT : Inport  Port=2  OutDataType=fixdt(1, 16)  OutScaling=2^0
  CLR_IRPT : Inport  Port=3  OutDataType=fixdt(1, 16)  OutScaling=2^0
  Delay : xbsIndex_r4/Delay  en=off  latency=1  dbl_ovrd=off  reg_retiming=off  block_type=delay
      settings: block_version=12.1
  Logical1 : xbsIndex_r4/Logical  logical_function=OR  inputs=2  en=off  latency=0  precision=Full  arith_type=Unsigned  n_bits=16  bin_pt=0  align_bp=on  dbl_ovrd=off  block_type=logical
      settings: block_version=12.1
  Logical2 : xbsIndex_r4/Logical  logical_function=XOR  inputs=2  en=off  latency=0  precision=Full  arith_type=Unsigned  n_bits=16  bin_pt=0  align_bp=on  dbl_ovrd=off  block_type=logical
      settings: block_version=12.1
  Logical4 : xbsIndex_r4/Logical  logical_function=AND  inputs=2  en=off  latency=0  precision=Full  arith_type=Unsigned  n_bits=16  bin_pt=0  align_bp=on  dbl_ovrd=off  block_type=logical
      settings: block_version=12.1
  Register : xbsIndex_r4/Register  init=0  rst=on  en=off  dbl_ovrd=off  block_type=register
      settings: block_version=12.1
  IRPT_OUT : Outport  OutDataType=fixdt(1, 16)  OutScaling=2^0
  wires:
  Delay/1 -> Logical2/2
  DIN/1 -> Delay/1, Logical2/1
  Logical2/1 -> Logical4/1
  EN_IRPT/1 -> Logical4/2
  Logical4/1 -> Logical1/2
  Logical1/1 -> Register/1
  Register/1 -> IRPT_OUT/1, Logical1/1
  CLR_IRPT/1 -> Register/2

== system Xcvr_SSB_AM_2p5/Serial Interface1/Interrupt_Generator/IRPT_REG2 ==
  DIN : Inport  OutDataType=fixdt(1, 16)  OutScaling=2^0
  EN_IRPT : Inport  Port=2  OutDataType=fixdt(1, 16)  OutScaling=2^0
  CLR_IRPT : Inport  Port=3  OutDataType=fixdt(1, 16)  OutScaling=2^0
  Delay : xbsIndex_r4/Delay  en=off  latency=1  dbl_ovrd=off  reg_retiming=off  block_type=delay
      settings: block_version=12.1
  Logical1 : xbsIndex_r4/Logical  logical_function=OR  inputs=2  en=off  latency=0  precision=Full  arith_type=Unsigned  n_bits=16  bin_pt=0  align_bp=on  dbl_ovrd=off  block_type=logical
      settings: block_version=12.1
  Logical2 : xbsIndex_r4/Logical  logical_function=XOR  inputs=2  en=off  latency=0  precision=Full  arith_type=Unsigned  n_bits=16  bin_pt=0  align_bp=on  dbl_ovrd=off  block_type=logical
      settings: block_version=12.1
  Logical4 : xbsIndex_r4/Logical  logical_function=AND  inputs=2  en=off  latency=0  precision=Full  arith_type=Unsigned  n_bits=16  bin_pt=0  align_bp=on  dbl_ovrd=off  block_type=logical
      settings: block_version=12.1
  Register : xbsIndex_r4/Register  init=0  rst=on  en=off  dbl_ovrd=off  block_type=register
      settings: block_version=12.1
  IRPT_OUT : Outport  OutDataType=fixdt(1, 16)  OutScaling=2^0
  wires:
  Delay/1 -> Logical2/2
  DIN/1 -> Delay/1, Logical2/1
  Logical2/1 -> Logical4/1
  EN_IRPT/1 -> Logical4/2
  Logical4/1 -> Logical1/2
  Logical1/1 -> Register/1
  Register/1 -> IRPT_OUT/1, Logical1/1
  CLR_IRPT/1 -> Register/2

== system Xcvr_SSB_AM_2p5/Serial Interface1/Interrupt_Generator/IRPT_REG3 ==
  DIN : Inport  OutDataType=fixdt(1, 16)  OutScaling=2^0
  EN_IRPT : Inport  Port=2  OutDataType=fixdt(1, 16)  OutScaling=2^0
  CLR_IRPT : Inport  Port=3  OutDataType=fixdt(1, 16)  OutScaling=2^0
  Delay : xbsIndex_r4/Delay  en=off  latency=1  dbl_ovrd=off  reg_retiming=off  block_type=delay
      settings: block_version=12.1
  Logical1 : xbsIndex_r4/Logical  logical_function=OR  inputs=2  en=off  latency=0  precision=Full  arith_type=Unsigned  n_bits=16  bin_pt=0  align_bp=on  dbl_ovrd=off  block_type=logical
      settings: block_version=12.1
  Logical2 : xbsIndex_r4/Logical  logical_function=XOR  inputs=2  en=off  latency=0  precision=Full  arith_type=Unsigned  n_bits=16  bin_pt=0  align_bp=on  dbl_ovrd=off  block_type=logical
      settings: block_version=12.1
  Logical4 : xbsIndex_r4/Logical  logical_function=AND  inputs=2  en=off  latency=0  precision=Full  arith_type=Unsigned  n_bits=16  bin_pt=0  align_bp=on  dbl_ovrd=off  block_type=logical
      settings: block_version=12.1
  Register : xbsIndex_r4/Register  init=0  rst=on  en=off  dbl_ovrd=off  block_type=register
      settings: block_version=12.1
  IRPT_OUT : Outport  OutDataType=fixdt(1, 16)  OutScaling=2^0
  wires:
  Delay/1 -> Logical2/2
  DIN/1 -> Delay/1, Logical2/1
  Logical2/1 -> Logical4/1
  EN_IRPT/1 -> Logical4/2
  Logical4/1 -> Logical1/2
  Logical1/1 -> Register/1
  Register/1 -> IRPT_OUT/1, Logical1/1
  CLR_IRPT/1 -> Register/2

== system Xcvr_SSB_AM_2p5/Serial Interface1/Interrupt_Generator/IRPT_REG4 ==
  note: K6JCA -- fpga test pin
  DIN : Inport  OutDataType=fixdt(1, 16)  OutScaling=2^0
  EN_IRPT : Inport  Port=2  OutDataType=fixdt(1, 16)  OutScaling=2^0
  CLR_IRPT : Inport  Port=3  OutDataType=fixdt(1, 16)  OutScaling=2^0
  Delay : xbsIndex_r4/Delay  en=off  latency=1  dbl_ovrd=off  reg_retiming=off  block_type=delay
      settings: block_version=12.1
  Logical1 : xbsIndex_r4/Logical  logical_function=OR  inputs=2  en=off  latency=0  precision=Full  arith_type=Unsigned  n_bits=16  bin_pt=0  align_bp=on  dbl_ovrd=off  block_type=logical
      settings: block_version=12.1
  Logical2 : xbsIndex_r4/Logical  logical_function=XOR  inputs=2  en=off  latency=0  precision=Full  arith_type=Unsigned  n_bits=16  bin_pt=0  align_bp=on  dbl_ovrd=off  block_type=logical
      settings: block_version=12.1
  Logical4 : xbsIndex_r4/Logical  logical_function=AND  inputs=2  en=off  latency=0  precision=Full  arith_type=Unsigned  n_bits=16  bin_pt=0  align_bp=on  dbl_ovrd=off  block_type=logical
      settings: block_version=12.1
  Register : xbsIndex_r4/Register  init=0  rst=on  en=off  dbl_ovrd=off  block_type=register
      settings: block_version=12.1
  IRPT_OUT : Outport  OutDataType=fixdt(1, 16)  OutScaling=2^0
  wires:
  Delay/1 -> Logical2/2
  DIN/1 -> Delay/1, Logical2/1
  Logical2/1 -> Logical4/1
  EN_IRPT/1 -> Logical4/2
  Logical4/1 -> Logical1/2
  Logical1/1 -> Register/1
  Register/1 -> IRPT_OUT/1, Logical1/1
  CLR_IRPT/1 -> Register/2

== system Xcvr_SSB_AM_2p5/Serial Interface1/Serial_in_Parallel_out/Serial2Par ==
  Sin : Inport
  ena : Inport  Port=2
  Concat : xbsIndex_r4/Concat  num_inputs=4  dbl_ovrd=off  block_type=concat
      settings: block_version=9.2.00
  Subsystem : Subsystem
  Subsystem1 : Subsystem
  Subsystem2 : Subsystem
  Subsystem3 : Subsystem
  Terminator : Terminator
  out_32b : Outport
  wires:
  Sin/1 -> Subsystem/1(Sin)
  ena/1 -> Subsystem/2(Ena), Subsystem1/2(Ena), Subsystem3/2(Ena), Subsystem2/2(Ena)
  Subsystem/2(Sout) -> Subsystem1/1(Sin)
  Subsystem1/2(Sout) -> Subsystem2/1(Sin)
  Subsystem2/2(Sout) -> Subsystem3/1(Sin)
  Concat/1 -> out_32b/1
  Subsystem3/1(Out_8b) -> Concat/1
  Subsystem2/1(Out_8b) -> Concat/2
  Subsystem1/1(Out_8b) -> Concat/3
  Subsystem/1(Out_8b) -> Concat/4
  Subsystem3/2(Sout) -> Terminator/1

== system Xcvr_SSB_AM_2p5/Serial Interface1/Serial_in_Parallel_out/delta_1 ==
  In1 : Inport
  Inverter : xbsIndex_r4/Inverter  en=off  latency=0  dbl_ovrd=off  block_type=inv
      settings: block_version=9.2.00
  Logical : xbsIndex_r4/Logical  logical_function=AND  inputs=2  en=off  latency=0  precision=Full  arith_type=Unsigned  n_bits=16  bin_pt=0  align_bp=on  dbl_ovrd=off  block_type=logical
      settings: block_version=9.2.00
  Register : xbsIndex_r4/Register  init=0  rst=off  en=off  dbl_ovrd=off  block_type=register
      settings: block_version=9.2.00
  Out1 : Outport
  wires:
  Register/1 -> Inverter/1
  Inverter/1 -> Logical/2
  Logical/1 -> Out1/1
  In1/1 -> Register/1, Logical/1

== system Xcvr_SSB_AM_2p5/Serial Interface1/Serial_in_Parallel_out/delta_2 ==
  In1 : Inport
  Inverter : xbsIndex_r4/Inverter  en=off  latency=0  dbl_ovrd=off  block_type=inv
      settings: block_version=9.2.00
  Logical : xbsIndex_r4/Logical  logical_function=AND  inputs=2  en=off  latency=0  precision=Full  arith_type=Unsigned  n_bits=16  bin_pt=0  align_bp=on  dbl_ovrd=off  block_type=logical
      settings: block_version=9.2.00
  Register : xbsIndex_r4/Register  init=0  rst=off  en=off  dbl_ovrd=off  block_type=register
      settings: block_version=9.2.00
  Out1 : Outport
  wires:
  In1/1 -> Logical/1, Register/1
  Logical/1 -> Out1/1
  Inverter/1 -> Logical/2
  Register/1 -> Inverter/1

== system Xcvr_SSB_AM_2p5/TX Filters I=8192/Control/Stage_Control ==
  Concat : xbsIndex_r4/Concat  num_inputs=3  dbl_ovrd=off  block_type=concat
      settings: block_version=9.2.00
  Constant : xbsIndex_r4/Constant  arith_type=Boolean  const=0  n_bits=16  bin_pt=14  explicit_period=off  period=1  equ=P=C  opselect=C  inp2=PCIN>>17  opr=+  inp1=P  carry=CIN  dbl_ovrd=off  block_type=constant
      settings: block_version=9.2.00
  Counter : xbsIndex_r4/Counter  cnt_type=Free Running  cnt_to=Inf  operation=Up  start_count=0  cnt_by_val=1  arith_type=Unsigned  n_bits=7  bin_pt=0  load_pin=off  rst=off  en=off  explicit_period=on  period=64/Fs  dbl_ovrd=off  use_behavioral_HDL=off  implementation=Fabric  use_rpm=off  block_type=counter
      settings: block_version=9.2.00
  Logical : xbsIndex_r4/Logical  logical_function=OR  inputs=7  en=off  latency=0  precision=Full  arith_type=Unsigned  n_bits=16  bin_pt=0  align_bp=on  dbl_ovrd=off  block_type=logical
      settings: block_version=9.2.00
  Mux : xbsIndex_r4/Mux  inputs=8  en=off  latency=0  precision=User Defined  arith_type=Unsigned  n_bits=1  bin_pt=0  quantization=Truncate  overflow=Wrap  dbl_ovrd=off  block_type=mux
      settings: block_version=9.2.00
  Priority_Encoder : Subsystem
  bit_0 : xbsIndex_r4/Slice  nbits=1  boolean_output=on  mode=Lower Bit Location + Width  bit1=0  base1=MSB of Input  bit0=0  base0=LSB of Input  dbl_ovrd=off  block_type=slice
      settings: infoedit="Extracts a given range of bits from each input sample and presents it at the output.  The output type is ordinarily unsigned with binary point at zero, but can be Boolean when the slice is one bit wide.<P><P>Hardware notes: In hardware this block costs nothing."  block_version=9.2.00
  bit_1 : xbsIndex_r4/Slice  nbits=1  boolean_output=on  mode=Lower Bit Location + Width  bit1=0  base1=MSB of Input  bit0=1  base0=LSB of Input  dbl_ovrd=off  block_type=slice
      settings: infoedit="Extracts a given range of bits from each input sample and presents it at the output.  The output type is ordinarily unsigned with binary point at zero, but can be Boolean when the slice is one bit wide.<P><P>Hardware notes: In hardware this block costs nothing."  block_version=9.2.00
  bit_2 : xbsIndex_r4/Slice  nbits=1  boolean_output=on  mode=Lower Bit Location + Width  bit1=0  base1=MSB of Input  bit0=2  base0=LSB of Input  dbl_ovrd=off  block_type=slice
      settings: infoedit="Extracts a given range of bits from each input sample and presents it at the output.  The output type is ordinarily unsigned with binary point at zero, but can be Boolean when the slice is one bit wide.<P><P>Hardware notes: In hardware this block costs nothing."  block_version=9.2.00
  bit_3 : xbsIndex_r4/Slice  nbits=1  boolean_output=on  mode=Lower Bit Location + Width  bit1=0  base1=MSB of Input  bit0=3  base0=LSB of Input  dbl_ovrd=off  block_type=slice
      settings: infoedit="Extracts a given range of bits from each input sample and presents it at the output.  The output type is ordinarily unsigned with binary point at zero, but can be Boolean when the slice is one bit wide.<P><P>Hardware notes: In hardware this block costs nothing."  block_version=9.2.00
  bit_4 : xbsIndex_r4/Slice  nbits=1  boolean_output=on  mode=Lower Bit Location + Width  bit1=0  base1=MSB of Input  bit0=4  base0=LSB of Input  dbl_ovrd=off  block_type=slice
      settings: infoedit="Extracts a given range of bits from each input sample and presents it at the output.  The output type is ordinarily unsigned with binary point at zero, but can be Boolean when the slice is one bit wide.<P><P>Hardware notes: In hardware this block costs nothing."  block_version=9.2.00
  bit_5 : xbsIndex_r4/Slice  nbits=1  boolean_output=on  mode=Lower Bit Location + Width  bit1=0  base1=MSB of Input  bit0=5  base0=LSB of Input  dbl_ovrd=off  block_type=slice
      settings: infoedit="Extracts a given range of bits from each input sample and presents it at the output.  The output type is ordinarily unsigned with binary point at zero, but can be Boolean when the slice is one bit wide.<P><P>Hardware notes: In hardware this block costs nothing."  block_version=9.2.00
  bit_6 : xbsIndex_r4/Slice  nbits=1  boolean_output=on  mode=Lower Bit Location + Width  bit1=0  base1=MSB of Input  bit0=6  base0=LSB of Input  dbl_ovrd=off  block_type=slice
      settings: infoedit="Extracts a given range of bits from each input sample and presents it at the output.  The output type is ordinarily unsigned with binary point at zero, but can be Boolean when the slice is one bit wide.<P><P>Hardware notes: In hardware this block costs nothing."  block_version=9.2.00
  Write_OK : Outport
  Filt_Stage : Outport  Port=2
  AB_Sel : Outport  Port=3
  wires:
  Concat/1 -> Filt_Stage/1, Mux/1  "Filt_Stage"
  Logical/1 -> Write_OK/1  "Write_OK"
  Priority_Encoder/3(Out3) -> Concat/1
  Priority_Encoder/1(Out1) -> Concat/3
  Priority_Encoder/2(Out2) -> Concat/2
  Counter/1 -> bit_5/1, bit_4/1, bit_3/1, bit_2/1, bit_1/1, bit_0/1, bit_6/1
  bit_6/1 -> Priority_Encoder/1(In1), Logical/1, Mux/7
  bit_5/1 -> Priority_Encoder/2(In2), Logical/2, Mux/6
  bit_4/1 -> Priority_Encoder/3(In3), Logical/3, Mux/5
  bit_3/1 -> Priority_Encoder/4(In4), Logical/4, Mux/4
  bit_2/1 -> Priority_Encoder/5(In5), Logical/5, Mux/3
  bit_1/1 -> Priority_Encoder/6(In6), Logical/6, Mux/2
  bit_0/1 -> Logical/7, Priority_Encoder/7(In7)
  Mux/1 -> AB_Sel/1
  Constant/1 -> Mux/9, Mux/8

== system Xcvr_SSB_AM_2p5/TX Filters I=8192/Interp_Core/RAM Based SR ==
  Xn_In : Inport
  Yn_in : Inport  Port=2
  Zn_in : Inport  Port=3
  Addr : Inport  Port=4
  En : Inport  Port=5
  Extend_Sign : Inport  Port=6
  4 bit Counter : xbsIndex_r4/Counter  cnt_type=Free Running  cnt_to=Inf  operation=Up  start_count=0  cnt_by_val=1  arith_type=Unsigned  n_bits=4  bin_pt=0  load_pin=off  rst=off  en=on  explicit_period=off  period=1  dbl_ovrd=off  use_behavioral_HDL=off  implementation=Fabric  use_rpm=off  block_type=counter
      settings: block_version=9.2.00
  Bit-Extraction : Subsystem
  BitBasher : xbsIndex_r4/BitBasher  bitexpr=|  display_expr=off  sr_1=1  arith_type1=Unsigned  bin_pt1=0  sr_2=2  arith_type2=Unsigned  bin_pt2=0  sr_3=3  arith_type3=Unsigned  bin_pt3=0  sr_4=4  arith_type4=Unsigned  bin_pt4=0  dbl_ovrd=off  block_type=bitbasher
      | <html><head><meta name="qrichtext" content="1" /></head><body style="font-size:8pt;font-family:MS Shell Dlg">
      | <p>a={b5,b4,b3,b2,b1,b0}</p>
      | </body></html>
      settings: block_version=9.2.00
      settings: infoedit=|
      | Allows
      |      extraction, concatenation and augmentation of bits
  Concat : xbsIndex_r4/Concat  num_inputs=2  dbl_ovrd=off  block_type=concat
      settings: block_version=9.2.00
  Single Port RAM : xbsIndex_r4/Single Port RAM  depth=256  initVector=zeros(1,256)  distributed_mem=Distributed memory  write_mode=Read Before Write  rst=off  init_reg=0  en=off  latency=0  dbl_ovrd=off  optimize=Area  use_rpm=on  block_type=spram
      settings: block_version=9.2.00
  Track and Hold k6jca : Subsystem
  Xn : Outport
  Xn-1 : Outport  Port=2
  Xn-2 : Outport  Port=3
  Xn-3 : Outport  Port=4
  Xn-4 : Outport  Port=5
  Yn-1 : Outport  Port=6
  Yn-2 : Outport  Port=7
  Zn-1 : Outport  Port=8
  Zn-2 : Outport  Port=9
  wires:
  BitBasher/1 -> Single Port RAM/2
  Xn_In/1 -> BitBasher/1, Track and Hold k6jca/1(In1)
  Addr/1 -> Concat/1
  4 bit Counter/1 -> Concat/2
  Concat/1 -> Single Port RAM/1
  Bit-Extraction/1(b0) -> BitBasher/2, Track and Hold k6jca/2(In2)
  Bit-Extraction/2(b1) -> BitBasher/3, Track and Hold k6jca/3(In3)
  Bit-Extraction/3(b2) -> BitBasher/4, Track and Hold k6jca/4(In4)
  Yn_in/1 -> BitBasher/5, Track and Hold k6jca/8(In8)
  Zn_in/1 -> BitBasher/6, Track and Hold k6jca/9(In9)
  En/1 -> 4 bit Counter/1, Single Port RAM/3
  Single Port RAM/1 -> Bit-Extraction/1(In1)
  Track and Hold k6jca/9(Out9) -> Zn-1/1
  Track and Hold k6jca/8(Out8) -> Yn-1/1
  Track and Hold k6jca/7(Out7) -> Zn-2/1
  Track and Hold k6jca/6(Out6) -> Yn-2/1
  Track and Hold k6jca/5(Out5) -> Xn-4/1
  Track and Hold k6jca/4(Out4) -> Xn-3/1
  Track and Hold k6jca/3(Out3) -> Xn-2/1
  Track and Hold k6jca/2(Out2) -> Xn-1/1
  Track and Hold k6jca/1(Out1) -> Xn/1
  Bit-Extraction/4(b3) -> Track and Hold k6jca/5(In5)
  Bit-Extraction/5(b4) -> Track and Hold k6jca/6(In6)
  Bit-Extraction/6(b5) -> Track and Hold k6jca/7(In7)
  Extend_Sign/1 -> Track and Hold k6jca/10(Extend_Sign)
